simulink model "NN__fault_detection_data_generator"  (R2018b)
settings: Solver=VariableStepAuto  StartTime=0.0  StopTime=0.05  RelTol=1e-3
undefined symbols (not defined in the file or in its folder): FT, s1_set, s2_set, s3_set, s4_set
libraries: powerlib x6, powerlib_meascontrol x1
settings Model: Creator=cy5924je  LastModifiedBy=samue
settings DataIOCC: ReturnWorkspaceOutputs=on

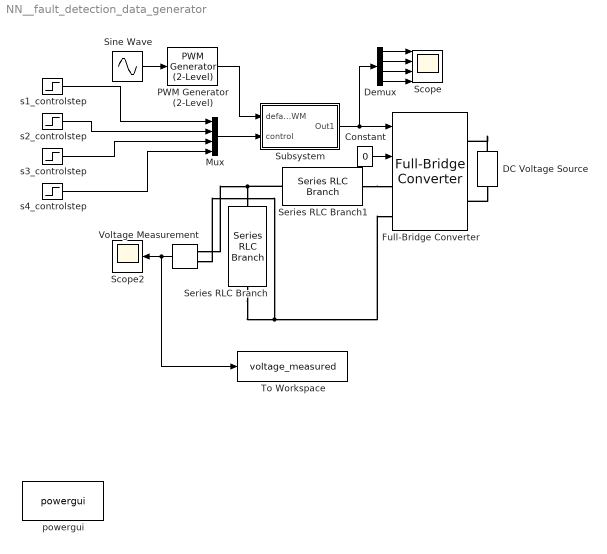
== system NN__fault_detection_data_generator ==
  Constant : Constant  Value=0
  DC Voltage Source : powerlib/Electrical Sources/DC Voltage Source  Amplitude=20  Measurements=None
      settings: SourceProductName=Simscape Electrical
  Demux : Demux
  Full-Bridge Converter : powerlib/Power Electronics/Full-Bridge Converter  ModelType=Switching devices  Ron=1e-3  Rs=1e6  Cs=inf  Vforward=[0,0]  Ron_Diode=1e-3  Rs_Diode=1e6  Cs_Diode=inf  Vf_Diode=1e-3  Rs_CurrentSource=inf
      settings: SourceProductName=Simscape Electrical  SourceProductBaseCode=PS
  Mux : Mux
  PWM Generator (2-Level) : powerlib_meascontrol/Pulse & Signal Generators/PWM Generator (2-Level)  ModulatorType=Single-phase full-bridge (4 pulses)  ModulatorMode=Unsynchronized  Fc=27*60  Pc=90  nF=27  MinMax="[ -1  1 ]"  SamplingTechnique=Natural  ModulatingSignals=off  m=0.8  Freq=60  Phase=0  Ts=0  ShowCarrierOutport=off
  Scope : Scope  NumInputPorts=4
  Scope2 : Scope
  Series RLC Branch : powerlib/Elements/Series RLC Branch  LConnTagsString=__new0  RConnTagsString=__new0  BranchType=RLC  Resistance=1  Inductance=0  SetiL0=off  InitialCurrent=0  Capacitance=0  Setx0=off  InitialVoltage=0  Measurements=None
      settings: SourceProductName=Simscape Electrical
  Series RLC Branch1 : powerlib/Elements/Series RLC Branch  LConnTagsString=__new0  RConnTagsString=__new0  BranchType=RLC  Resistance=1  Inductance=1e-3  SetiL0=off  InitialCurrent=0  Capacitance=0  Setx0=off  InitialVoltage=0  Measurements=None
      settings: SourceProductName=Simscape Electrical
  Sine Wave : Sin  Frequency=377  SampleTime=0
  Subsystem : Subsystem
  To Workspace : ToWorkspace  VariableName=voltage_measured  SaveFormat=Timeseries  SampleTime=-1
  Voltage Measurement : powerlib/Measurements/Voltage Measurement  PhasorSimulation=off  OutputType=Complex  PSBequivalent=0
      settings: SourceProductName=Simscape Electrical
  powergui : powerlib/powergui  Priority=1  SimulationMode=Continuous  SampleTime=50e-6  frequency=60  Iterations=50  frequencyindice=0  Pbase=100e6  ErrMax=1e-4  UnitsV=kV  UnitsW=MW  buscounter=0  FunctionMessages=off  echomessages=off  EnableUseOfTLC=off  CurrentSourceSwitches=off  DisableSnubberDevices=off  DisableRonSwitches=off  DisableVfSwitches=off  DisplayEquations=off  AutomaticDiscreteSolvers=off  SolverType=Tustin/Backward Euler (TBE)  Interpol=off  ExternalGateDelay=off  methode=off  Ts=100  x0status=blocks  SPID=on  SwTol=0  HookPort=off  NonlinearTolerance=0  nMaxIteration=15  ContinueOnMaxIteration=off  RestoreLinks=warning  ResistiveCurrentMeasurement=off  Frange=[0:2:500]  Ylog=off  Xlog=on  ShowGrid=off  save=off  variable=ZData  structure=0  ZoomFFT=off  StartTime=0.0  cycles=1  DisplayStyle=1  fundamental=60  FreqAxis=off  MaxFrequency=1000  frequencyindicesteady=1  RmsSteady=1  display=off
      settings: SourceProductName=Simscape Electrical
  s1_controlstep : Step  Time=FT  Before=2  After=s1_set  SampleTime=0
  s2_controlstep : Step  Time=FT  Before=2  After=s2_set  SampleTime=0
  s3_controlstep : Step  Time=FT  Before=2  After=s3_set  SampleTime=0
  s4_controlstep : Step  Time=FT  Before=2  After=s4_set  SampleTime=0
  wires:
  Constant/1 -> Full-Bridge Converter/2
  Sine Wave/1 -> PWM Generator (2-Level)/1
  Voltage Measurement/1 -> To Workspace/1, Scope2/1
  Demux/1 -> Scope/1
  Demux/2 -> Scope/2
  Demux/3 -> Scope/3
  Demux/4 -> Scope/4
  PWM Generator (2-Level)/1 -> Subsystem/1(default_PWM)
  Subsystem/1(Out1) -> Demux/1, Full-Bridge Converter/1
  Mux/1 -> Subsystem/2(control)
  s1_controlstep/1 -> Mux/1
  s4_controlstep/1 -> Mux/4
  s3_controlstep/1 -> Mux/3
  s2_controlstep/1 -> Mux/2
  connections:
  DC Voltage Source/RConn1 -- Full-Bridge Converter/RConn1
  DC Voltage Source/LConn1 -- Full-Bridge Converter/RConn2
  Voltage Measurement/LConn1 -- Series RLC Branch/LConn1 -- Series RLC Branch1/LConn1
  Voltage Measurement/LConn2 -- Series RLC Branch/RConn1 -- Full-Bridge Converter/LConn2
  Series RLC Branch1/RConn1 -- Full-Bridge Converter/LConn1

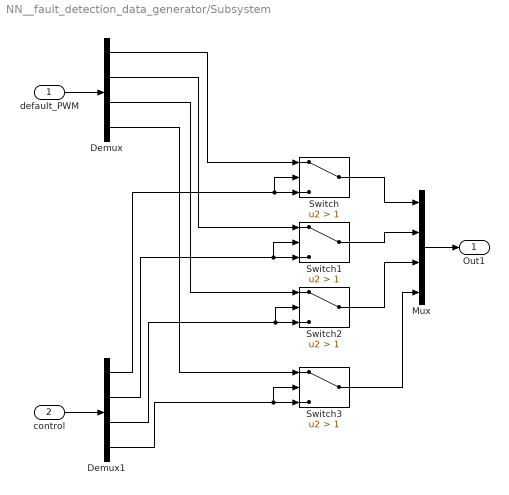
== system NN__fault_detection_data_generator/Subsystem ==
  default_PWM : Inport
  control : Inport  Port=2
  Demux : Demux
  Demux1 : Demux
  Mux : Mux
  Switch{,1..3} (4 alike) : Switch  Criteria=u2 > Threshold  Threshold=1
  Out1 : Outport  VectorParamsAs1DForOutWhenUnconnected=off
  wires:
  default_PWM/1 -> Demux/1
  Mux/1 -> Out1/1
  Demux1/3 -> Switch2/2, Switch2/3
  control/1 -> Demux1/1
  Demux1/4 -> Switch3/2, Switch3/3
  Demux1/2 -> Switch1/2, Switch1/3
  Demux1/1 -> Switch/2, Switch/3
  Demux/1 -> Switch/1
  Demux/2 -> Switch1/1
  Demux/3 -> Switch2/1
  Demux/4 -> Switch3/1
  Switch/1 -> Mux/1
  Switch1/1 -> Mux/2
  Switch2/1 -> Mux/3
  Switch3/1 -> Mux/4
